simulink model "Heavy_duty_AC_Motor_R2020a"  (R2020a)
settings: Solver=VariableStepAuto  StartTime=0.0  StopTime=60*60*8  RelTol=1e-3
values from neighbouring files (symbols this model uses):
  Rotor_inertia = 1.4    [Parameters.m]
libraries: nesl_utility x9, fl_lib x4, simulink x1, ee_lib x1
settings Model: Creator=YXL1108  LastModifiedBy=YXL1108

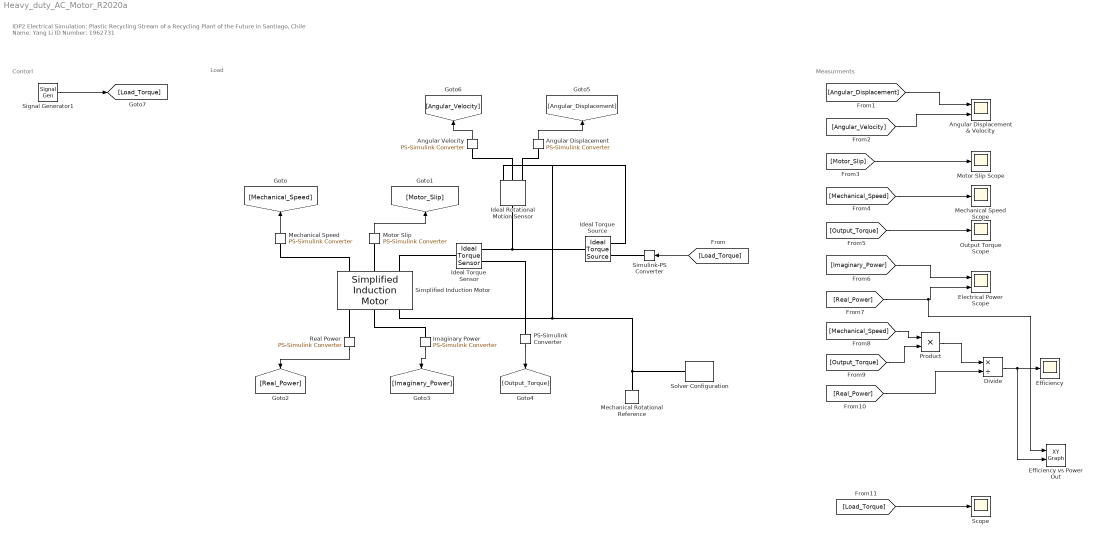
== system Heavy_duty_AC_Motor_R2020a ==
  note: Measurments
  note: Contorl
  note: Load
  note: IDP2 Electrical Simulation: Plastic Recycling Stream of a Recycling Plant of the Future in Santiago, Chile
      | Name: Yang Li
      | ID Number: 1962731
  Angular Displacement : nesl_utility/PS-Simulink Converter  PhysicalDomain=network_engine_domain  SubClassName=ps_output  LeftPortType=input  RightPortType=output  PseudoPeriodic=off  Frequencies=[]  Unit=inherit  AffineConversion=off
  Angular Displacement & Velocity : Scope  NumInputPorts=2
  Angular Velocity : nesl_utility/PS-Simulink Converter  PhysicalDomain=network_engine_domain  SubClassName=ps_output  LeftPortType=input  RightPortType=output  PseudoPeriodic=off  Frequencies=[]  Unit=inherit  AffineConversion=off
  Divide : Product  Inputs=*/
  Efficiency : Scope
  Efficiency vs Power Out : simulink/Sinks/XY Graph  xmin=-300  xmax=60000  ymin=0  ymax=5  st=-1
  Electrical Power Scope : Scope  NumInputPorts=2
  Ideal Rotational Motion Sensor : fl_lib/Mechanical/Mechanical Sensors/Ideal Rotational Motion Sensor  wrap_angle=simscape.enum.onoff.off  offset=0 rad
  Ideal Torque Sensor : fl_lib/Mechanical/Mechanical Sensors/Ideal Torque Sensor
  Ideal Torque Source : fl_lib/Mechanical/Mechanical Sources/Ideal Torque Source
  Imaginary Power : nesl_utility/PS-Simulink Converter  PhysicalDomain=network_engine_domain  SubClassName=ps_output  LeftPortType=input  RightPortType=output  PseudoPeriodic=off  Frequencies=[]  Unit=inherit  AffineConversion=off
  Mechanical Rotational Reference : fl_lib/Mechanical/Rotational Elements/Mechanical Rotational Reference
  Mechanical Speed : nesl_utility/PS-Simulink Converter  PhysicalDomain=network_engine_domain  SubClassName=ps_output  LeftPortType=input  RightPortType=output  PseudoPeriodic=off  Frequencies=[]  Unit=inherit  AffineConversion=off
  Mechanical Speed Scope : Scope
  Motor Slip : nesl_utility/PS-Simulink Converter  PhysicalDomain=network_engine_domain  SubClassName=ps_output  LeftPortType=input  RightPortType=output  PseudoPeriodic=off  Frequencies=[]  Unit=inherit  AffineConversion=off
  Motor Slip Scope : Scope
  Output Torque Scope : Scope
  PS-Simulink Converter : nesl_utility/PS-Simulink Converter  PhysicalDomain=network_engine_domain  SubClassName=ps_output  LeftPortType=input  RightPortType=output  PseudoPeriodic=off  Frequencies=[]  Unit=inherit  AffineConversion=off
  Product : Product
  Real Power : nesl_utility/PS-Simulink Converter  PhysicalDomain=network_engine_domain  SubClassName=ps_output  LeftPortType=input  RightPortType=output  PseudoPeriodic=off  Frequencies=[]  Unit=inherit  AffineConversion=off
  Scope : Scope
  Signal Generator1 : SignalGenerator  WaveForm=square  Amplitude=10  Units=rad/sec
  Simplified Induction Motor : ee_lib/Electromechanical/Asynchronous/Simplified Induction Motor  param=1  R1=1 Ohm  R2=1 Ohm  L1=0.02 H  L2=0.02 H  Lm=0.5 H  P_rated=Rated_mechanical_power kW  w_mech=Rated_speed rpm  v_rated=Rated_RMS_line_to_line_voltage V  w_rated=Rated_supply_frequency Hz  i_rated=Rated_RMS_line_current A  paramR1=1  E=Motor_efficiency_percent  pf=0.93  R1m=1 Ohm  V=Supply_RMS_line_to_line_voltage V  w=Supply_frequency Hz  p=Number_of_pole_pairs  n=Number_of_phases  paramLoad=2  J=Rotor_inertia kg*m^2  lam=Rotor_damping N*m/(rad/s)  speed0=Initial_rotor_speed rpm  alpha=[.00393, .00393] 1/K  Tmeas=25 degC  thermal_masses=[100, 100] J/K  initial_temperatures=[25, 25] degC
      settings: SourceProductBaseCode=PS  InternalSimscapePortConfiguration="{\"Bottom\":[],\"Left\":[{\"id\":\"wm\",\"label\":\"wm\",\"type\":\"output\"},{\"id\":\"slip\",\"label\":\"s\",\"type\":\"output\"},{\"id\":\"R\",\"label\":\"R\",\"type\":\"foundation.mechanical.rotational.rotational\"}],\"Right\":[{\"id\":\"Watts\",\"label\":\"W\",\"type\":\"output\"},{\"id\":\"VARs\",\"label\":\"VAR\",\"type\":\"output\"},{\"id\":\"C\",\"label\":\"C\",\"type\":\"foundation.mechanical.rotational.rotational\"}],\"Top\":[]}"
  Simulink-PS Converter : nesl_utility/Simulink-PS Converter  PhysicalDomain=network_engine_domain  SubClassName=ps_input  LeftPortType=input  RightPortType=output  PseudoPeriodic=off  Frequencies=[]  NoiseDistribution=none  NoiseParameters=[]  Unit=1  AffineConversion=off  FilteringAndDerivatives=provide  SimscapeFilterOrder=1  InputFilterTimeConstant=0.001  UdotUserProvided=0
  Solver Configuration : nesl_utility/Solver Configuration  PhysicalDomain=network_engine_domain  SubClassName=solver  LeftPortType=input  RightPortType=generic  Tones=[]  Harmonics=[]  SimulateNoise=off  Profile=off  UseLocalSampling=off  EnableSwitchedLinearOptims=on  FrequencyDomain=off  UseCCode=off  RelTol=0.001  AbsTol=1e-06  MinStep=1e-09  ToWorkspace=off  RevertToSquareIcSolve=off  NumHomotopyIterations=100  PhasorMode=off  PhasorModeNumHarmonics=1  DoDC=off  ResidualTolerance=1e-09  UseLocalSolver=off  LocalSolverChoice=NE_BACKWARD_EULER_ADVANCER  LocalSolverSampleTime=0.001  DoFixedCost=off  MaxNonlinIter=3  MaxModeIter=2  LinearAlgebra=auto  EquationFormulation=NE_TIME_EF  DelaysMemoryBudget=1024  AutomaticFiltering=on  FilteringTimeConstant=0.001  PartitionStorageMethod=AS_NEEDED  PartitionMemoryBudget=1024  PartitionMethod=ROBUST
  wires:
  Mechanical Speed/1 -> [Mechanical_Speed]
  Motor Slip/1 -> [Motor_Slip]
  Real Power/1 -> [Real_Power]
  Imaginary Power/1 -> [Imaginary_Power]
  PS-Simulink Converter/1 -> [Output_Torque]
  [Load_Torque] -> Simulink-PS Converter/1
  Angular Displacement/1 -> [Angular_Displacement]
  Angular Velocity/1 -> [Angular_Velocity]
  [Angular_Displacement] -> Angular Displacement & Velocity/1
  [Angular_Velocity] -> Angular Displacement & Velocity/2
  [Imaginary_Power] -> Electrical Power Scope/1
  [Real_Power] -> Efficiency vs Power Out/1, Electrical Power Scope/2
  [Mechanical_Speed] -> Mechanical Speed Scope/1
  [Motor_Slip] -> Motor Slip Scope/1
  [Output_Torque] -> Output Torque Scope/1
  Signal Generator1/1 -> [Load_Torque]
  [Output_Torque] -> Product/2
  [Mechanical_Speed] -> Product/1
  Product/1 -> Divide/1
  [Real_Power] -> Divide/2
  Divide/1 -> Efficiency vs Power Out/2, Efficiency/1
  [Load_Torque] -> Scope/1
  connections:
  Mechanical Speed/LConn1 -- Simplified Induction Motor/LConn1
  Motor Slip/LConn1 -- Simplified Induction Motor/LConn2
  Real Power/LConn1 -- Simplified Induction Motor/RConn1
  Imaginary Power/LConn1 -- Simplified Induction Motor/RConn2
  Simplified Induction Motor/RConn3 -- Ideal Torque Source/RConn2 -- Ideal Rotational Motion Sensor/RConn1 -- Solver Configuration/RConn1 -- Mechanical Rotational Reference/LConn1
  Simplified Induction Motor/LConn3 -- Ideal Torque Sensor/LConn1
  Ideal Torque Sensor/RConn1 -- Ideal Torque Source/LConn1 -- Ideal Rotational Motion Sensor/LConn1
  Ideal Torque Sensor/RConn2 -- PS-Simulink Converter/LConn1
  Simulink-PS Converter/RConn1 -- Ideal Torque Source/RConn1
  Ideal Rotational Motion Sensor/RConn2 -- Angular Velocity/LConn1
  Ideal Rotational Motion Sensor/RConn3 -- Angular Displacement/LConn1
